simulink model "controller_stateflow"  (R2022b)
settings: Solver=FixedStepAuto  StartTime=0.0  StopTime=inf  FixedStep=0.05  RelTol=1e-3
PreLoadFcn:
  | rosinit();
model workspace (MAT data in the model file):
  SL_ROS_VariableLengthArrays_MaxSizes : object (value not decoded)
  pitch = -10
  restart = 0
undefined symbols (not defined in the file): StartTime
libraries: robotmaniplib x62, robotlib x17, robotcorelib x4, robotgazebolib x1
(part 4 of 4)

== stateflow chart controller_stateflow/General State Flow ==
  state Initialization0 [group]
    state initial_state
      entry:
      fprintf("Simulation started, setting initial conditions... ");
      sum_pos = [0;0;0];
      sum_ZYX = [0;0;0];
      send_command_ur10e = 0;
      send_command_panda = 0;
      send_command_sum = 0;
      panda_durTime = 2;
      ur_durTime = 2;
      state_velvet = 0;
      hand_state = 0.2;
      state_4 = 0;
      state_4_collBox = state_4;
      if pick_type<4
      state_4 = 2;
      end
    state initial_pose
      entry: fprintf("\n Go to home position...");
      [ur_pos,ur_durTime] = set_ur_initialState1();
      [panda_pos,panda_durTime] = set_panda_initialState();
      during:
      send_command_ur10e = 1;
      send_command_panda = 1;
      send_command_sum = 1;
    state Ready
      during: fprintf("--> Home position and initial poses done! \n");
      send_command_ur10e = 0;
      send_command_panda = 0;
      send_command_sum = 0;
      hand_state = 0.2;
    Initialization0.initial_state -> Initialization0.initial_pose : [controller_ready && link_state_ready]
    Initialization0.initial_pose -> Initialization0.Ready : [ur_finish && panda_finish && sum_finish]
  state Initialization [group]
    state initial_state
      entry:
      fprintf("Simulation started, setting initial conditions... ");
      sum_pos = [0;0;0];
      sum_ZYX = [0;0;0];
      send_command_ur10e = 0;
      send_command_panda = 0;
      send_command_sum = 0;
      panda_durTime = 2;
      ur_durTime = 2;
      state_velvet = 0;
      hand_state = 0.2;
      state_4 = 0;
      state_4_collBox = state_4;
      if pick_type<4
      state_4 = 2;
      end
    state initial_pose
      entry: fprintf("\n Go to home position...");
      [ur_pos,ur_durTime] = set_ur_initialState();
      [panda_pos,panda_durTime] = set_panda_initialState();
      during:
      send_command_ur10e = 1;
      send_command_panda = 1;
      send_command_sum = 1;
    state Ready
      entry: fprintf("--> Home position and initial poses done! \n");
      send_command_ur10e = 0;
      send_command_panda = 0;
      send_command_sum = 0;
      hand_state = 0.2;
    Initialization.initial_state -> Initialization.initial_pose : [controller_ready && link_state_ready]
    Initialization.initial_pose -> Initialization.Ready : [ur_finish && panda_finish && sum_finish]
  state [ur_pos,ur_durTime] = get_ur_pose4(box_pos,box_ZYX,box2_pos,box2_ZYX,sum_actual_pos,sum_actual_ZYX,ur_state,state) [function]
  state [ur_pos,durTime_ur] = get_ur_pose3(box_pose,box_ZYX,sum_actual_pos,sum_actual_ZYX,ur_state,state) [function]
  state [ur_pos,durTime_ur] = get_ur_pose(box_pose,box_ZYX,sum_actual_pos,sum_actual_ZYX,ur_state,state) [function]
  state [ur_pos,durTime_ur] = get_ur_pose2(box_pose,box_ZYX,sum_actual_pos,sum_actual_ZYX,ur_state,state) [function]
  state [panda_pos, panda_durTime] = get_panda_pose4(box_pos,box_ZYX,box2_pos,box2_ZYX,sum_actual_pos,sum_actual_ZYX,panda_state,state) [function]
  state [panda_pos,durTime_panda] = get_panda_pose3(box_pos,box_ZYX,sum_actual_pos,sum_actual_ZYX,panda_state,state) [function]
  state [panda_pos,durTime_panda] = get_panda_pose(box_pos,box_ZYX,sum_actual_pos,sum_actual_ZYX,panda_state,state) [function]
  state [panda_pos,durTime_panda] = get_panda_pose2(box_pos,box_ZYX,sum_actual_pos,sum_actual_ZYX,panda_state,state) [function]
  state Primitive_1 [group]
    state Going_near_the_pallet
      entry:
      fprintf("Picking type : 1 \n");
      fprintf("State 1: Going near the pallet... \n");
      during:
      distance_from_box = 0.8;
      distance_10 = 0.2;
      [sum_pos,sum_ZYX] = get_sum_pose_from_box(box_pos,box_ZYX,distance_from_box,distance_10,pick_type);
      send_command_sum = 1;
    state Setting_initial_arms_poses
      entry: fprintf("State 2: Setting initial arms poses... ");
      send_command_ur10e = 0;
      send_command_panda = 0;
      send_command_sum = 0;
      [ur_pos,ur_durTime] = get_ur_pose(box_pos,box_ZYX,sum_actual_pos,sum_actual_ZYX,ur_state,2);
      [panda_pos, panda_durTime] = get_panda_pose(box_pos,box_ZYX,sum_actual_pos,sum_actual_ZYX,panda_state,2);
      during:
      send_command_ur10e=1;
      send_command_panda = 1;
    state Going_near_the_box
      entry:fprintf("State 3: Going near the box... \n");
      send_command_panda = 0;
      send_command_sum = 0;
      distance_10 = 0;
      during:
      [sum_pos,sum_ZYX] = get_sum_pose_from_box(box_pos,box_ZYX,distance_from_box,distance_10,pick_type);
      send_command_sum = 1;
    state Softhand_goes_down
      entry: fprintf("State 4: Softhand goes down...\n");
      send_command_ur10e = 0;
      send_command_panda = 0;
      send_command_sum = 0;
      [ur_pos,ur_durTime] = get_ur_pose(box_pos,box_ZYX,sum_actual_pos,sum_actual_ZYX,ur_state,4);
      [panda_pos, panda_durTime]  = get_panda_pose(box_pos,box_ZYX,sum_actual_pos,sum_actual_ZYX,panda_state,4);
      during:
      send_command_panda = 1;
      send_command_ur10e = 1;
    state Getting_box_on_velvet
      entry: fprintf("State 5: Getting box on velvet...\n");
      send_command_panda = 0;
      send_command_ur10e = 0;
      [panda_pos, panda_durTime]  = get_panda_pose(box_pos,box_ZYX,sum_actual_pos,sum_actual_ZYX,panda_state,5);
      during:
      send_command_panda = 1;
      state_velvet = 1; %pick-up
    state Going_back_from_the_pallet_and_setting_holding_box_arms_poses
      entry: fprintf("State 7: Going back from the pallet...\n");
      fprintf("Setting holding box arms poses... ");
      distance_from_box = 0.8;
      distance_10 = 0.3;
      [sum_pos,sum_ZYX] = get_sum_pose_from_box(box_pos,box_ZYX,distance_from_box,distance_10,pick_type);
      send_command_ur10e = 0;
      send_command_panda = 0;
      send_command_sum = 0;
      [ur_pos,ur_durTime] = get_ur_pose(box_pos,box_ZYX,sum_actual_pos,sum_actual_ZYX,ur_state,7);
      [panda_pos, panda_durTime] = get_panda_pose(box_pos,box_ZYX,sum_actual_pos,sum_actual_ZYX,panda_state,7);
      during:
      send_command_sum = 1;
      send_command_ur10e=1;
      send_command_panda = 1;
    Primitive_1.Going_near_the_pallet -> Primitive_1.Setting_initial_arms_poses : [sum_finish && go>=2]
    Primitive_1.Setting_initial_arms_poses -> Primitive_1.Going_near_the_box : [ur_finish && panda_finish && go>=3]
    Primitive_1.Going_near_the_box -> Primitive_1.Softhand_goes_down : [sum_finish && go>=4]
    Primitive_1.Softhand_goes_down -> Primitive_1.Getting_box_on_velvet : [ur_finish && panda_finish && go>=5]{hand_state = 0.4;}
    Primitive_1.Getting_box_on_velvet -> Primitive_1.Going_back_from_the_pallet_and_setting_holding_box_arms_poses : [panda_finish && box_on_velvet && go>=6]{state_velvet = 0;}
  state Primitive_2 [group]
    state Going_near_the_pallet
      entry:
      fprintf("Picking type : 2 \n");
      fprintf("State 1: Going near the pallet... \n");
      during:
      distance_from_box = 0.85;
      distance_10 = 0.2;
      [sum_pos,sum_ZYX] = get_sum_pose_from_box(box_pos,box_ZYX,distance_from_box,distance_10,pick_type);
      send_command_sum = 1;
    state Setting_initial_arms_poses
      entry: fprintf("State 2: Setting initial arms poses... ");
      send_command_ur10e = 0;
      send_command_panda = 0;
      send_command_sum = 0;
      [ur_pos,ur_durTime] = get_ur_pose2(box_pos,box_ZYX,sum_actual_pos,sum_actual_ZYX,ur_state,2);
      [panda_pos, panda_durTime] = get_panda_pose2(box_pos,box_ZYX,sum_actual_pos,sum_actual_ZYX,panda_state,2);
      during:
      send_command_ur10e=1;
      send_command_panda = 1;
    state Going_near_the_box
      entry:fprintf("State 3: Going near the box... \n");
      send_command_panda = 0;
      send_command_sum = 0;
      distance_10 = 0;
      during:
      [sum_pos,sum_ZYX] = get_sum_pose_from_box(box_pos,box_ZYX,distance_from_box,distance_10,pick_type);
      send_command_sum = 1;
    state Softhand_goes_down
      entry: fprintf("State 4: Softhand goes down...\n");
      send_command_ur10e = 0;
      send_command_panda = 0;
      send_command_sum = 0;
      [panda_pos, panda_durTime]  = get_panda_pose2(box_pos,box_ZYX,sum_actual_pos,sum_actual_ZYX,panda_state,4);
      during:
      send_command_panda = 1;
    state Close_hand_and_approach_edge
      entry: fprintf("State 5: Close hand and approach edge...\n");
      send_command_panda = 0;
      hand_state = 0.6;
      [panda_pos, panda_durTime]  = get_panda_pose2(box_pos,box_ZYX,sum_actual_pos,sum_actual_ZYX,panda_state,5);
      during:
      send_command_panda = 1;
    state Getting_box_on_velvet
      entry: fprintf("State 6: Getting box on velvet...\n");
      send_command_panda = 0;
      [panda_pos, panda_durTime]  = get_panda_pose2(box_pos,box_ZYX,sum_actual_pos,sum_actual_ZYX,panda_state,6);
      during:
      send_command_panda = 1;
      %state_velvet = 1; %pick-up
    state Hand_up
      entry: fprintf("State 7: Hand up...\n");
      send_command_ur10e = 0;
      send_command_panda = 0;
      send_command_sum = 0;
      hand_state = 0.2;
      send_command_panda = 0;
      [panda_pos, panda_durTime]  = get_panda_pose2(box_pos,box_ZYX,sum_actual_pos,sum_actual_ZYX,panda_state,7);
      during:
      send_command_panda = 1;
    state Hand_reaches_the_lower_edge
      entry: fprintf("State 8: Hand reaches the lower edge...\n");
      send_command_panda = 0;
      [panda_pos, panda_durTime]  = get_panda_pose2(box_pos,box_ZYX,sum_actual_pos,sum_actual_ZYX,panda_state,8);
      during:
      send_command_panda = 1;
    state Hand_approaches_the_lower_edge
      entry: fprintf("State 9: Hand approaches the lower edge...\n");
      send_command_panda = 0;
      [panda_pos, panda_durTime]  = get_panda_pose2(box_pos,box_ZYX,sum_actual_pos,sum_actual_ZYX,panda_state,9);
      during:
      send_command_panda = 1;
    state Getting_the_box_aligned
      entry:
      entry: fprintf("State 10: Getting the box aligned...\n");
      send_command_ur10e = 0;
      send_command_panda = 0;
      send_command_sum = 0;
      sum_pos = sum_pos - [0;0.25;0];
      [ur_pos,ur_durTime] = get_ur_pose2(box_pos,box_ZYX,sum_actual_pos,sum_actual_ZYX,ur_state,10);
      [panda_pos, panda_durTime]  = get_panda_pose2(box_pos,box_ZYX,sum_actual_pos,sum_actual_ZYX,panda_state,10);
      during:
      send_command_ur10e=1;
      send_command_panda = 1;
      send_command_sum = 1;
    state Hand_approaches_the_lower_edge1
      entry: fprintf("State 11: Hand approaches the lower edge...\n");
      send_command_ur10e = 0;
      send_command_panda = 0;
      [panda_pos, panda_durTime]  = get_panda_pose2(box_pos,box_ZYX,sum_actual_pos,sum_actual_ZYX,panda_state,11);
      during:
      send_command_panda = 1;
    state Going_back_from_the_pallet_and_setting_holding_box_arms_poses
      entry: fprintf("State 12: Going back from the pallet...\n");
      fprintf("Settin holding box arms poses... ");
      distance_from_box = 0.8;
      distance_10 = 0.3;
      %[sum_pos,sum_ZYX] = get_sum_pose_from_box(box_pos,box_ZYX,distance_from_box,distance_10,pick_type);
      sum_pos = sum_pos - [0;0.5;0];
      send_command_ur10e = 0;
      send_command_panda = 0;
      send_command_sum = 0;
      [ur_pos,ur_durTime] = get_ur_pose(box_pos,box_ZYX,sum_actual_pos,sum_actual_ZYX,ur_state,7);
      [panda_pos, panda_durTime] = get_panda_pose(box_pos,box_ZYX,sum_actual_pos,sum_actual_ZYX,panda_state,7);
      during:
      send_command_sum = 1;
      send_command_ur10e=1;
      send_command_panda = 1;
    Primitive_2.Going_near_the_pallet -> Primitive_2.Setting_initial_arms_poses : [sum_finish && go>=2]
    Primitive_2.Setting_initial_arms_poses -> Primitive_2.Going_near_the_box : [ur_finish && panda_finish && go>=3]
    Primitive_2.Going_near_the_box -> Primitive_2.Softhand_goes_down : [sum_finish && go>=4]
    Primitive_2.Softhand_goes_down -> Close_hand_and_approach_edge : [panda_finish && go>=5]
    Close_hand_and_approach_edge -> Primitive_2.Getting_box_on_velvet : [panda_finish && go>=6]
    Primitive_2.Getting_box_on_velvet -> Hand_up : [panda_finish && box_on_velvet && go>=7]{state_velvet = 0;}
    Hand_up -> Hand_reaches_the_lower_edge : [panda_finish && go>=8]
    Hand_reaches_the_lower_edge -> Hand_approaches_the_lower_edge : [panda_finish && go>=9]
    Hand_approaches_the_lower_edge -> Getting_the_box_aligned : [panda_finish && go>=10]{hand_state = 0.6;}
    Getting_the_box_aligned -> Hand_approaches_the_lower_edge1 : [ur_finish && panda_finish && go>=11]{hand_state = 0.2;}
    Hand_approaches_the_lower_edge1 -> Primitive_2.Going_back_from_the_pallet_and_setting_holding_box_arms_poses : [panda_finish && go>=12]
  state Primitive_3 [group]
    state Going_near_the_pallet
      entry:
      fprintf("Picking type : 3 \n");
      fprintf("State 1: Going near the pallet... \n");
      during:
      distance_from_box = 0.85;
      distance_10 = 0.2;
      [sum_pos,sum_ZYX] = get_sum_pose_from_box(box_pos,box_ZYX,distance_from_box,distance_10,pick_type);
      send_command_sum = 1;
    state Setting_initial_arms_poses
      entry: fprintf("State 2: Setting initial arms poses... \n");
      send_command_ur10e = 0;
      send_command_panda = 0;
      send_command_sum = 0;
      [ur_pos,ur_durTime] = get_ur_pose3(box_pos,box_ZYX,sum_actual_pos,sum_actual_ZYX,ur_state,2);
      [panda_pos, panda_durTime] = get_panda_pose3(box_pos,box_ZYX,sum_actual_pos,sum_actual_ZYX,panda_state,2);
      during:
      send_command_ur10e=1;
      send_command_panda = 1;
    state Going_near_the_box
      entry:fprintf("State 3: Going near the box... \n");
      send_command_panda = 0;
      send_command_sum = 0;
      distance_10 = 0;
      during:
      [sum_pos,sum_ZYX] = get_sum_pose_from_box(box_pos,box_ZYX,distance_from_box,distance_10,pick_type);
      send_command_sum = 1;
    state Setting_initial_arms_poses_nearly
      entry: fprintf("State 4: Setting initial arms poses nearly... \n ");
      send_command_ur10e = 0;
      send_command_panda = 0;
      send_command_sum = 0;
      [ur_pos,ur_durTime] = get_ur_pose3(box_pos,box_ZYX,sum_actual_pos,sum_actual_ZYX,ur_state,4);
      [panda_pos, panda_durTime] = get_panda_pose3(box_pos,box_ZYX,sum_actual_pos,sum_actual_ZYX,panda_state,4);
      during:
      send_command_ur10e=1;
      send_command_panda = 1;
    state Softhand_goes_down
      entry: fprintf("State 5: Sofhand goes down...\n");
      send_command_ur10e = 0;
      send_command_panda = 0;
      [panda_pos, panda_durTime]  = get_panda_pose3(box_pos,box_ZYX,sum_actual_pos,sum_actual_ZYX,panda_state,5);
      during:
      send_command_panda = 1;
    state Softhand_reanches_and_approaches_the_edge
      entry: fprintf("State 6: Softhand reanches and approaches the edge, box up... \n");
      send_command_panda = 0;
      hand_state = 0.6;
      [panda_pos, panda_durTime]  = get_panda_pose3(box_pos,box_ZYX,sum_actual_pos,sum_actual_ZYX,panda_state,6);
      during:
      send_command_panda = 1;
    state Moving_Velvet_towards_the_box
      entry: fprintf("State 7: Moving Velvet towards the box... ");
      send_command_panda = 0;
      [ur_pos,ur_durTime] = get_ur_pose3(box_pos,box_ZYX,sum_actual_pos,sum_actual_ZYX,ur_state,7);
      during:
      send_command_ur10e = 1;
    state Moving_Velvet_under_the_box
      entry: fprintf("State 8: Moving Velvet under the box... ");
      send_command_ur10e = 0;
      [ur_pos,ur_durTime] = get_ur_pose3(box_pos,box_ZYX,sum_actual_pos,sum_actual_ZYX,ur_state,8);
      during:
      send_command_ur10e = 1;
    state Softhand_goes_far_from_box
      entry: fprintf("State 9: Softhand goes far from box...\n");
      send_command_panda = 0;
      send_command_ur10e = 0;
      [panda_pos, panda_durTime]  = get_panda_pose3(box_pos,box_ZYX,sum_actual_pos,sum_actual_ZYX,panda_state,9);
      during:
      send_command_panda = 1;
    state Getting_box_on_velvet
      entry: fprintf("State 10: Getting box on velvet, velvet on \n ");
      send_command_panda = 0;
      during:
      state_velvet = 1; %pick-up
    state Going_back_from_the_pallet_and_setting_holding_box_arms_poses
      entry: fprintf("State 11: Going back from the pallet...\n");
      fprintf("Settin holding box arms poses... ");
      distance_from_box = 1;
      distance_10 = 0.3;
      [sum_pos,sum_ZYX] = get_sum_pose_from_box(box_pos,box_ZYX,distance_from_box,distance_10,pick_type);
      send_command_ur10e = 0;
      send_command_panda = 0;
      send_command_sum = 0;
      [ur_pos,ur_durTime] = get_ur_pose3(box_pos,box_ZYX,sum_actual_pos,sum_actual_ZYX,ur_state,11);
      %[panda_pos, panda_durTime] = get_panda_pose3(box_pos,box_ZYX,sum_actual_pos,sum_actual_ZYX,panda_state,11);
      during:
      send_command_sum = 1;
      send_command_ur10e=1;
      %send_command_panda = 1;
    state Sofhand_goes_down
      entry: fprintf("State 12: Sofhand goes down ...\n");
      send_command_panda = 0;
      send_command_ur10e = 0;
      send_command_sum = 0;
      [panda_pos, panda_durTime]  = get_panda_pose3(box_pos,box_ZYX,sum_actual_pos,sum_actual_ZYX,panda_state,12);
      during:
      send_command_panda = 1;
    state Softhand_holding_box
      entry: fprintf("State 13: Sofhand holding box... \n");
      send_command_panda = 0;
      send_command_ur10e = 0;
      send_command_sum = 0;
      [panda_pos, panda_durTime]  = get_panda_pose3(box_pos,box_ZYX,sum_actual_pos,sum_actual_ZYX,panda_state,13);
      during:
      send_command_panda = 1;
      exit: hand_state = 0.4;
    Primitive_3.Going_near_the_pallet -> Primitive_3.Setting_initial_arms_poses : [sum_finish && go>=2]
    Primitive_3.Setting_initial_arms_poses -> Primitive_3.Going_near_the_box : [ur_finish && panda_finish && go>=3]
    Primitive_3.Going_near_the_box -> Setting_initial_arms_poses_nearly : [sum_finish && go>=4]
    Setting_initial_arms_poses_nearly -> Primitive_3.Softhand_goes_down : [ur_finish && panda_finish && go>=5]
    Primitive_3.Softhand_goes_down -> Softhand_reanches_and_approaches_the_edge : [panda_finish && go>=6]
    Softhand_reanches_and_approaches_the_edge -> Moving_Velvet_towards_the_box : [panda_finish && go>=7]
    Moving_Velvet_towards_the_box -> Moving_Velvet_under_the_box : [ur_finish && go>= 8]
    Moving_Velvet_under_the_box -> Softhand_goes_far_from_box : [ur_finish && go>=9]{ hand_state = 0.2;}
    Softhand_goes_far_from_box -> Primitive_3.Getting_box_on_velvet : [panda_finish && go >=10]
    Primitive_3.Getting_box_on_velvet -> Primitive_3.Going_back_from_the_pallet_and_setting_holding_box_arms_poses : [box_on_velvet]{state_velvet = 0;}
    Primitive_3.Going_back_from_the_pallet_and_setting_holding_box_arms_poses -> Sofhand_goes_down : [ur_finish && go>=12]
    Sofhand_goes_down -> Softhand_holding_box : [panda_finish && go>=13]
  state Primitive_4 [group]
    state Going_near_the_pallet
      entry:
      fprintf("Picking type : 4 \n");
      fprintf("State 1: Going near the pallet... \n");
      during:
      distance_from_box = 0.8;
      distance_10 = 0.2;
      [sum_pos,sum_ZYX] = get_sum_pose_from_box4(box_pos,box_ZYX,box2_pos,box2_ZYX,distance_from_box,distance_10,state_4);
      send_command_sum = 1;
    state Open_both_hands2
      entry: fprintf("Picking Strategy for the second box. \n");
      fprintf("State 2: Open both hands... ");
      send_command_ur10e = 0;
      send_command_panda = 0;
      send_command_sum = 0;
      [ur_pos,ur_durTime] = get_ur_pose4(box_pos,box_ZYX,box2_pos,box2_ZYX,sum_actual_pos,sum_actual_ZYX,ur_state,102);
      [panda_pos, panda_durTime] = get_panda_pose4(box_pos,box_ZYX,box2_pos,box2_ZYX,sum_actual_pos,sum_actual_ZYX,panda_state,102);
      during:
      send_command_ur10e=1;
      send_command_panda = 1;
    state Open_both_hands
      entry: fprintf("Picking Strategy for the first box. \n");
      fprintf("State 2: Open both hands... ");
      send_command_ur10e = 0;
      send_command_panda = 0;
      send_command_sum = 0;
      [ur_pos,ur_durTime] = get_ur_pose4(box_pos,box_ZYX,box2_pos,box2_ZYX,sum_actual_pos,sum_actual_ZYX,ur_state,101);
      [panda_pos, panda_durTime] = get_panda_pose4(box_pos,box_ZYX,box2_pos,box2_ZYX,sum_actual_pos,sum_actual_ZYX,panda_state,101);
      during:
      send_command_ur10e=1;
      send_command_panda = 1;
    state Going_near_the_box2
      entry:fprintf("State 3: Going near the box... \n");
      distance_10 = 0;
      during:
      [sum_pos,sum_ZYX] = get_sum_pose_from_box4(box_pos,box_ZYX,box2_pos,box2_ZYX,distance_from_box,distance_10,state_4);
      send_command_sum = 1;
    state Going_near_the_box
      entry:fprintf("State 3: Going near the box... \n");
      distance_10 = 0;
      during:
      [sum_pos,sum_ZYX] = get_sum_pose_from_box4(box_pos,box_ZYX,box2_pos,box2_ZYX,distance_from_box,distance_10,state_4);
      send_command_sum = 1;
    state Hold_both_boxes
      entry: fprintf("State 4: Hold both boxes... ");
      send_command_ur10e = 0;
      send_command_panda = 0;
      send_command_sum = 0;
      [ur_pos,ur_durTime] = get_ur_pose4(box_pos,box_ZYX,box2_pos,box2_ZYX,sum_actual_pos,sum_actual_ZYX,ur_state,111);
      [panda_pos, panda_durTime] = get_panda_pose4(box_pos,box_ZYX,box2_pos,box2_ZYX,sum_actual_pos,sum_actual_ZYX,panda_state,111);
      during:
      send_command_ur10e=1;
      send_command_panda = 1;
    state Hold_both_boxes2
      entry: fprintf("State 4: Hold both boxes... ");
      send_command_ur10e = 0;
      send_command_panda = 0;
      send_command_sum = 0;
      [ur_pos,ur_durTime] = get_ur_pose4(box_pos,box_ZYX,box2_pos,box2_ZYX,sum_actual_pos,sum_actual_ZYX,ur_state,112);
      [panda_pos, panda_durTime] = get_panda_pose4(box_pos,box_ZYX,box2_pos,box2_ZYX,sum_actual_pos,sum_actual_ZYX,panda_state,112);
      during:
      send_command_ur10e=1;
      send_command_panda = 1;
    state Rotate_first_box
      entry: fprintf("State 5: Rotate first box... ");
      send_command_ur10e = 0;
      send_command_panda = 0;
      [panda_pos, panda_durTime]  = get_panda_pose4(box_pos,box_ZYX,box2_pos,box2_ZYX,sum_actual_pos,sum_actual_ZYX,panda_state,121);
      during:
      send_command_panda = 1;
    state Rotate_second_box
      entry: fprintf("State 5: Rotate second box... ");
      send_command_panda = 0;
      send_command_ur10e = 0;
      hand_state = 0.5;
      [ur_pos,ur_durTime] = get_ur_pose4(box_pos,box_ZYX,box2_pos,box2_ZYX,sum_actual_pos,sum_actual_ZYX,ur_state,122);
      [panda_pos, panda_durTime]  = get_panda_pose4(box_pos,box_ZYX,box2_pos,box2_ZYX,sum_actual_pos,sum_actual_ZYX,panda_state,122);
      during:
      send_command_panda = 1;
      send_command_ur10e = 1;
    state Reopen_both_arms1
      entry: fprintf("State 6: Reopen both arms.. ");
      send_command_panda = 0;
      send_command_ur10e = 0;
      hand_state = 0.2;
      [ur_pos,ur_durTime] = get_ur_pose4(box_pos,box_ZYX,box2_pos,box2_ZYX,sum_actual_pos,sum_actual_ZYX,ur_state,132);
      [panda_pos, panda_durTime]  = get_panda_pose4(box_pos,box_ZYX,box2_pos,box2_ZYX,sum_actual_pos,sum_actual_ZYX,panda_state,132);
      during:
      send_command_panda = 1;
      send_command_ur10e=1;
    state Reopen_both_arms
      entry: fprintf("State 6: Reopen both arms.. ");
      send_command_panda = 0;
      send_command_ur10e = 0;
      [ur_pos,ur_durTime] = get_ur_pose4(box_pos,box_ZYX,box2_pos,box2_ZYX,sum_actual_pos,sum_actual_ZYX,ur_state,131);
      [panda_pos, panda_durTime]  = get_panda_pose4(box_pos,box_ZYX,box2_pos,box2_ZYX,sum_actual_pos,sum_actual_ZYX,panda_state,131);
      during:
      send_command_panda = 1;
      send_command_ur10e=1;
    Primitive_4.Going_near_the_pallet -> Open_both_hands [order 1] : [sum_finish && state_4 == 1 && go>=2]
    Primitive_4.Going_near_the_pallet -> Open_both_hands2 [order 2] : [sum_finish && state_4 == 2 && go>=2]
    Open_both_hands2 -> Going_near_the_box2 : [ur_finish && panda_finish && go>=3]
    Open_both_hands -> Primitive_4.Going_near_the_box : [ur_finish && panda_finish && go>=3]
    Primitive_4.Going_near_the_box -> Hold_both_boxes : [sum_finish && go>=4]
    Going_near_the_box2 -> Hold_both_boxes2 : [sum_finish && go>=4]
    Hold_both_boxes -> Rotate_first_box : [ur_finish && panda_finish && go>=5]
    Hold_both_boxes2 -> Rotate_second_box : [ur_finish && panda_finish && go>=5]
    Rotate_first_box -> Reopen_both_arms : [panda_finish && go>=6]
    Rotate_second_box -> Reopen_both_arms1 : [ur_finish && panda_finish && go>=6]
  state Primitive_1_for_piking_type_4 [group]
    state Going_near_the_pallet
      entry:
      fprintf("Picking type : 1 \n");
      fprintf("State 1: Going near the pallet... \n");
      during:
      distance_from_box = 0.8;
      distance_10 = 0.2;
      [sum_pos,sum_ZYX] = get_sum_pose_from_box(box_pos,box_ZYX,distance_from_box,distance_10,pick_type);
      send_command_sum = 1;
    state Going_near_the_pallet1
      entry:
      fprintf("Picking type : 1 \n");
      fprintf("State 1: Going near the pallet... \n");
      during:
      distance_from_box = 0.8;
      distance_10 = 0.2;
      [sum_pos,sum_ZYX] = get_sum_pose_from_box(box2_pos,box2_ZYX,distance_from_box,distance_10,pick_type);
      send_command_sum = 1;
    state Setting_initial_arms_poses
      entry: fprintf("State 2: Setting initial arms poses... ");
      send_command_ur10e = 0;
      send_command_panda = 0;
      send_command_sum = 0;
      [ur_pos,ur_durTime] = get_ur_pose(box_pos,box_ZYX,sum_actual_pos,sum_actual_ZYX,ur_state,2);
      [panda_pos, panda_durTime] = get_panda_pose(box_pos,box_ZYX,sum_actual_pos,sum_actual_ZYX,panda_state,2);
      during:
      send_command_ur10e=1;
      send_command_panda = 1;
    state Setting_initial_arms_poses1
      entry: fprintf("State 2: Setting initial arms poses... ");
      send_command_ur10e = 0;
      send_command_panda = 0;
      send_command_sum = 0;
      [ur_pos,ur_durTime] = get_ur_pose(box2_pos,box2_ZYX,sum_actual_pos,sum_actual_ZYX,ur_state,2);
      [panda_pos, panda_durTime] = get_panda_pose(box2_pos,box2_ZYX,sum_actual_pos,sum_actual_ZYX,panda_state,2);
      during:
      send_command_ur10e=1;
      send_command_panda = 1;
    state Going_near_the_box
      entry:fprintf("State 3: Going near the box... \n");
      send_command_panda = 0;
      send_command_sum = 0;
      distance_10 = 0;
      during:
      [sum_pos,sum_ZYX] = get_sum_pose_from_box(box_pos,box_ZYX,distance_from_box,distance_10,pick_type);
      send_command_sum = 1;
    state Going_near_the_box1
      entry:fprintf("State 3: Going near the box... \n");
      send_command_panda = 0;
      send_command_sum = 0;
      distance_10 = 0;
      during:
      [sum_pos,sum_ZYX] = get_sum_pose_from_box(box2_pos,box2_ZYX,distance_from_box,distance_10,pick_type);
      send_command_sum = 1;
    state Softhand_goes_down
      entry: fprintf("State 4: Softhand goes down...\n");
      send_command_ur10e = 0;
      send_command_panda = 0;
      send_command_sum = 0;
      [ur_pos,ur_durTime] = get_ur_pose(box_pos,box_ZYX,sum_actual_pos,sum_actual_ZYX,ur_state,4);
      [panda_pos, panda_durTime]  = get_panda_pose(box_pos,box_ZYX,sum_actual_pos,sum_actual_ZYX,panda_state,4);
      during:
      send_command_panda = 1;
      send_command_ur10e = 1;
    state Softhand_goes_down1
      entry: fprintf("State 4: Softhand goes down...\n");
      send_command_ur10e = 0;
      send_command_panda = 0;
      send_command_sum = 0;
      [ur_pos,ur_durTime] = get_ur_pose(box2_pos,box2_ZYX,sum_actual_pos,sum_actual_ZYX,ur_state,4);
      [panda_pos, panda_durTime]  = get_panda_pose(box2_pos,box2_ZYX,sum_actual_pos,sum_actual_ZYX,panda_state,4);
      during:
      send_command_panda = 1;
      send_command_ur10e = 1;
    state Getting_box_on_velvet
      entry: fprintf("State 5: Getting box on velvet...\n");
      send_command_panda = 0;
      send_command_ur10e = 0;
      [panda_pos, panda_durTime]  = get_panda_pose(box_pos,box_ZYX,sum_actual_pos,sum_actual_ZYX,panda_state,5);
      during:
      send_command_panda = 1;
      state_velvet = 1; %pick-up
    state Getting_box_on_velvet1
      entry: fprintf("State 5: Getting box on velvet...\n");
      send_command_panda = 0;
      send_command_ur10e = 0;
      [panda_pos, panda_durTime]  = get_panda_pose(box2_pos,box2_ZYX,sum_actual_pos,sum_actual_ZYX,panda_state,5);
      during:
      send_command_panda = 1;
      state_velvet = 1; %pick-up
    state Hold_box_on_velvet
      entry: fprintf("State 6: Hold box on velvet...\n");
      send_command_panda = 0;
      [panda_pos, panda_durTime]  = get_panda_pose(box_pos,box_ZYX,sum_actual_pos,sum_actual_ZYX,panda_state,6);
      during:
      send_command_panda = 1;
    state Hold_box_on_velvet1
      entry: fprintf("State 6: Hold box on velvet...\n");
      send_command_panda = 0;
      [panda_pos, panda_durTime]  = get_panda_pose(box2_pos,box2_ZYX,sum_actual_pos,sum_actual_ZYX,panda_state,6);
      during:
      send_command_panda = 1;
    state Going_back_from_the_pallet_and_setting_holding_box_arms_poses
      entry: fprintf("State 7: Going back from the pallet...\n");
      fprintf("Setting holding box arms poses... ");
      distance_from_box = 0.8;
      distance_10 = 0.3;
      [sum_pos,sum_ZYX] = get_sum_pose_from_box(box_pos,box_ZYX,distance_from_box,distance_10,pick_type);
      send_command_ur10e = 0;
      send_command_panda = 0;
      send_command_sum = 0;
      [ur_pos,ur_durTime] = get_ur_pose(box_pos,box_ZYX,sum_actual_pos,sum_actual_ZYX,ur_state,7);
      [panda_pos, panda_durTime] = get_panda_pose(box_pos,box_ZYX,sum_actual_pos,sum_actual_ZYX,panda_state,7);
      during:
      send_command_sum = 1;
      send_command_ur10e=1;
      send_command_panda = 1;
    state Going_back_from_the_pallet_and_setting_holding_box_arms_poses1
      entry: fprintf("State 7: Going back from the pallet...\n");
      fprintf("Setting holding box arms poses... ");
      distance_from_box = 0.8;
      distance_10 = 0.3;
      [sum_pos,sum_ZYX] = get_sum_pose_from_box(box2_pos,box2_ZYX,distance_from_box,distance_10,pick_type);
      send_command_ur10e = 0;
      send_command_panda = 0;
      send_command_sum = 0;
      [ur_pos,ur_durTime] = get_ur_pose(box2_pos,box2_ZYX,sum_actual_pos,sum_actual_ZYX,ur_state,7);
      [panda_pos, panda_durTime] = get_panda_pose(box2_pos,box2_ZYX,sum_actual_pos,sum_actual_ZYX,panda_state,7);
      during:
      send_command_sum = 1;
      send_command_ur10e=1;
      send_command_panda = 1;
    Primitive_1_for_piking_type_4.Going_near_the_pallet -> Primitive_1_for_piking_type_4.Setting_initial_arms_poses : [sum_finish && go>=8]
    Going_near_the_pallet1 -> Setting_initial_arms_poses1 : [sum_finish && go>=8]
    Primitive_1_for_piking_type_4.Setting_initial_arms_poses -> Primitive_1_for_piking_type_4.Going_near_the_box : [ur_finish && panda_finish && go>=9]
    Setting_initial_arms_poses1 -> Going_near_the_box1 : [ur_finish && panda_finish && go>=9]
    Primitive_1_for_piking_type_4.Going_near_the_box -> Primitive_1_for_piking_type_4.Softhand_goes_down : [sum_finish && go>=10]
    Going_near_the_box1 -> Softhand_goes_down1 : [sum_finish && go>=10]
    Primitive_1_for_piking_type_4.Softhand_goes_down -> Primitive_1_for_piking_type_4.Getting_box_on_velvet : [ur_finish && panda_finish && go>=11]{hand_state = 0.4;}
    Softhand_goes_down1 -> Getting_box_on_velvet1 : [ur_finish && panda_finish && go>=11]{hand_state = 0.4;}
    Primitive_1_for_piking_type_4.Getting_box_on_velvet -> Primitive_1_for_piking_type_4.Going_back_from_the_pallet_and_setting_holding_box_arms_poses : [panda_finish && box_on_velvet && go>=12]{state_velvet = 0;}
    Getting_box_on_velvet1 -> Going_back_from_the_pallet_and_setting_holding_box_arms_poses1 : [panda_finish && box_on_velvet && go>=12]{state_velvet = 0;}
    Hold_box_on_velvet -> Primitive_1_for_piking_type_4.Going_back_from_the_pallet_and_setting_holding_box_arms_poses : [panda_finish && go>=13]
    Hold_box_on_velvet1 -> Going_back_from_the_pallet_and_setting_holding_box_arms_poses1 : [panda_finish && go>=13]
  state Return home with box [group]
    state Go_back
      entry: fprintf("Picking phase completed! \n");
      fprintf("Return home position... \n");
      send_command_sum = 0;
      send_command_ur10e = 0;
      send_command_panda = 0;
      during:
      sum_pos = [0;0;0];
      sum_ZYX = [0;0;0];
      send_command_sum = 1;
    state finish
      entry: fprintf("Home position reached...\n");
      send_command_sum = 0;
    Go_back -> Return.finish : [sum_finish]
  state [ur_pos,durTime_ur] = get_ur_pose_cnvy(tra_pos,tra_ZYX,sum_actual_pos,sum_actual_ZYX,ur_state,state) [function]
  state [panda_pos,durTime_panda] = get_panda_pose_cnvy(tra_pos,tra_ZYX,sum_actual_pos,sum_actual_ZYX,panda_state,state) [function]
  state Release [group]
    state Go_near_the_conveyor_belt
      entry : fprintf("Release Phase: \n");
      fprintf("Go near the conveyor belt ... \n");
      during:
      distance_from_cnvy = 0.8;
      [sum_pos,sum_ZYX] = get_sum_pose_from_cnvy(tra_pos,tra_ZYX,distance_from_cnvy);
      send_command_sum = 1;
    state Franka_Hand_up
      entry: fprintf("Franka Hand Up... \n");
      send_command_ur10e = 0;
      send_command_panda = 0;
      send_command_sum = 0;
      [panda_pos, panda_durTime] = get_panda_pose_cnvy(box_pos,box_ZYX,sum_actual_pos,sum_actual_ZYX,panda_state,93);
      during:
      send_command_panda = 1;
    state Align_UR_Velvet
      entry: fprintf("Align UR Velvet... \n");
      send_command_ur10e = 0;
      send_command_panda = 0;
      send_command_sum = 0;
      [ur_pos,ur_durTime] = get_ur_pose_cnvy(tra_pos,tra_ZYX,sum_actual_pos,sum_actual_ZYX,ur_state,1);
      during:
      send_command_ur10e = 1;
    state Pull_out_box
      entry: fprintf("Box Off... \n");
      during:
      state_velvet = -1; %pick-off
    state Go_back_from_the_conveyor_belt
      entry: fprintf("Release phase completed! \n");
      fprintf("Go back from the conveyor belt... \n");
      send_command_ur10e = 0;
      send_command_panda = 0;
      send_command_sum = 0;
      during:
      distance_from_cnvy = 0.8;
      [sum_pos,sum_ZYX] = get_sum_pose_from_cnvy(tra_pos,tra_ZYX,distance_from_cnvy);
      send_command_sum = 1;
    Go_near_the_conveyor_belt -> Franka_Hand_up : [sum_finish && go>21]
    Franka_Hand_up -> Align_UR_Velvet : [panda_finish && go>22]
    Align_UR_Velvet -> Pull_out_box : [ur_finish  && go>23]
    Pull_out_box -> Go_back_from_the_conveyor_belt : [box_off && go>24]{state_velvet = 0;}
  state Finish [group]
    state Return_home
      entry:
      fprintf("Return home position... \n");
      send_command_sum = 0;
      during:
      sum_pos = [0;0;0];
      sum_ZYX = [0;0;0];
      [ur_pos,ur_durTime] = set_ur_initialState();
      [panda_pos,panda_durTime] = set_panda_initialState();
      send_command_ur10e = 1;
      send_command_panda = 1;
      send_command_sum = 1;
    state finish
      entry: fprintf(" --- Mission Completed ! --- \n");
      send_command_ur10e = 0;
      send_command_panda = 0;
      send_command_sum = 0;
    Return_home -> Finish.finish : [ur_finish && panda_finish && sum_finish]
  state THE_END
  (default) -> Initialization0.initial_state
  Initialization0.Ready -> Initialization.initial_state : [go > 1]
  Go_back_from_the_conveyor_belt -> Initialization.initial_pose [order 1] : [sum_finish && go>16 && state_4 == 1]
  Initialization.Ready -> Primitive_4.Going_near_the_pallet [order 3] : [pick_type == 4 && go>=1]{state_4 = state_4 +1; state_4_collBox = state_4;}
  Initialization.Ready -> Primitive_1.Going_near_the_pallet [order 2] : [pick_type == 1 && go>=1]
  Initialization.Ready -> Primitive_2.Going_near_the_pallet [order 1] : [pick_type == 2 && go>=1]
  Initialization.Ready -> Primitive_3.Going_near_the_pallet [order 4] : [pick_type == 3 && go>=1]
  Reopen_both_arms -> Primitive_1_for_piking_type_4.Going_near_the_pallet : [ur_finish && panda_finish && go>=7]
  Reopen_both_arms1 -> Going_near_the_pallet1 : [ur_finish && panda_finish && go>=7]
  Primitive_1.Going_back_from_the_pallet_and_setting_holding_box_arms_poses -> Go_back : [sum_finish && go>=8]
  Primitive_2.Going_back_from_the_pallet_and_setting_holding_box_arms_poses -> Go_back : [sum_finish && go>=13]
  Softhand_holding_box -> Go_back : [panda_finish && go>=14]
  Primitive_1_for_piking_type_4.Going_back_from_the_pallet_and_setting_holding_box_arms_poses -> Go_back : [sum_finish && go>14]
  Going_back_from_the_pallet_and_setting_holding_box_arms_poses1 -> Go_back : [sum_finish && go>14]
  Return.finish -> Go_near_the_conveyor_belt : [go>20]
  Go_back_from_the_conveyor_belt -> Return_home [order 2] : [sum_finish && go>25 && state_4 == 2]
  Finish.finish -> THE_END
  data: ur_Pos function_output; ur_durTime_ function_output; ur_Pos function_output; ur_durTime_ function_output; panda_pos function_output; panda_durTime_ function_output; sum_pos function_output; sum_ZYX function_output; box_pos function_input; box_ZYX function_input; distance_from_box function_input; distance_10 function_input; pick_type function_input; sum_pos function_output; sum_ZYX function_output; box_pos function_input; box_ZYX function_input; box2_pos function_input; box2_ZYX function_input; distance_from_box function_input; distance_10 function_input; state_4 function_input; box_pos function_input double size=[3,1]; box_ZYX function_input double size=[3,1]; box2_pos function_input double size=[3,1]; box2_ZYX function_input double size=[3,1]; sum_actual_pos function_input double size=[3,1]; sum_actual_ZYX function_input double size=[3,1]; ur_state function_input double size=[7,1]; ur_pos function_output; ur_durTime function_output; state function_input double size=1; box_pose function_input double size=[3,1]; box_ZYX function_input double size=[3,1]; sum_actual_pos function_input double size=[3,1]; sum_actual_ZYX function_input double size=[3,1]; ur_state function_input double size=[7,1]; ur_pos function_output; state function_input double size=1; durTime_ur function_output; box_pose function_input double size=[3,1]; box_ZYX function_input double size=[3,1]; sum_actual_pos function_input double size=[3,1]; sum_actual_ZYX function_input double size=[3,1]; ur_state function_input double size=[7,1]; ur_pos function_output; state function_input double size=1; durTime_ur function_output; box_pose function_input double size=[3,1]; box_ZYX function_input double size=[3,1]; sum_actual_pos function_input double size=[3,1]; sum_actual_ZYX function_input double size=[3,1]; ur_state function_input double size=[7,1]; ur_pos function_output; state function_input double size=1; durTime_ur function_output; box_pos function_input double size=[3,1]; box_ZYX function_input double size=[3,1]; box2_pos function_input double size=[3,1]; box2_ZYX function_input double size=[3,1]; sum_actual_pos function_input double size=[3,1]; sum_actual_ZYX function_input double size=[3,1]; panda_state function_input double size=[7,1]; panda_pos function_output; panda_durTime function_output; state function_input double size=1; box_pos function_input double size=[3,1]; box_ZYX function_input double size=[3,1]; sum_actual_pos function_input double size=[3,1]; sum_actual_ZYX function_input double size=[3,1]; panda_state function_input double size=[7,1]; panda_pos function_output; state function_input double size=1; durTime_panda function_output; box_pos function_input double size=[3,1]; box_ZYX function_input double size=[3,1]; sum_actual_pos function_input double size=[3,1]; sum_actual_ZYX function_input double size=[3,1]; panda_state function_input double size=[7,1]; panda_pos function_output; state function_input double size=1; durTime_panda function_output; box_pos function_input double size=[3,1]; box_ZYX function_input double size=[3,1]; sum_actual_pos function_input double size=[3,1]; sum_actual_ZYX function_input double size=[3,1]; panda_state function_input double size=[7,1]; panda_pos function_output; state function_input double size=1; durTime_panda function_output; sum_pos function_output; sum_ZYX function_output; tra_pos function_input; tra_ZYX function_input; distance_from_cnvy function_input; tra_pos function_input double size=[3,1]; tra_ZYX function_input double size=[3,1]; sum_actual_pos function_input double size=[3,1]; sum_actual_ZYX function_input double size=[3,1]; ur_state function_input double size=[7,1]; state function_input double size=1; ur_pos function_output; durTime_ur function_output; tra_pos function_input double size=[3,1]; tra_ZYX function_input double size=[3,1]; sum_actual_pos function_input double size=[3,1]; sum_actual_ZYX function_input double size=[3,1]; panda_state function_input double size=[7,1]; panda_pos function_output; state function_input double size=1; durTime_panda function_output; sf_internal_action_state_placeholder_data local double size=1 =0; pick_type input; send_command_ur10e output size=1,1; controller_ready input; link_state_ready input; go input; send_command_panda output size=1,1; send_command_sum output size=1,1; ur_pos output size=[6,5]; ur_durTime output size=1; panda_pos output; panda_durTime output size=1; sum_pos output; panda_state input; ur_state input; sum_actual_pos input; sum_actual_ZYX input; panda_finish input; sum_finish input; ur_finish input; box_pos input; box_ZYX input; sum_ZYX output; distance_10 local; distance_from_box local; box_on_velvet input; box_off input; box2_pos input size=[3,1]; box2_ZYX input size=[3,1]; tra_ZYX input; tra_pos input; state_velvet output size=1; hand_state output; state_4 local; state_4_collBox output size=1; distance_from_cnvy local
  function [ur_Pos,ur_durTime_]= set_ur_initialState1:
    | function [ur_Pos,ur_durTime_]= set_ur_initialState1
    | % Set initial pose of UR Manipulator
    | 
    |     
    |     ur_pos_  = ([0 -90 0 0 0 0]').*pi/180;
    | 
    |     ur_Pos = horzcat(ur_pos_,ur_pos_,ur_pos_,ur_pos_,ur_pos_);
    |     ur_durTime_ = 3;
    | end
  function [ur_Pos,ur_durTime_]= set_ur_initialState:
    | function [ur_Pos,ur_durTime_]= set_ur_initialState
    | % Set initial pose of UR Manipulator
    | 
    |     ur_pos_  = [-0.6416,-5.6222+2*pi,-2.4013,-4.5429+2*pi,0.9292,-3.1416]';
    |     ur_pos_  = ([-90-71.37,-102.78,-141.66,-70.64,-62.79,-205.96]').*pi/180;
    | 
    |     ur_Pos = horzcat(ur_pos_,ur_pos_,ur_pos_,ur_pos_,ur_pos_);
    |     ur_durTime_ = 3;
    | end
  function [panda_pos,panda_durTime_] = set_panda_initialState:
    | function [panda_pos,panda_durTime_] = set_panda_initialState
    | % Set initial pose of Panda Manipulator
    |  panda_pos_ = [0;-0.7853;0;-2.35619;0;1.57079;0.785398];
    |  panda_pos = horzcat(panda_pos_,panda_pos_,panda_pos_,panda_pos_,panda_pos_);
    |  panda_durTime_ = 3;
    | end
  function [sum_pos,sum_ZYX] = get_sum_pose_from_box(box_pos,box_ZYX,distance_from_box,distance_10,pick_type):
    | function [sum_pos,sum_ZYX] = get_sum_pose_from_box(box_pos,box_ZYX,distance_from_box,distance_10,pick_type)
    |     
    |     base_sum_length = 0.75; 
    |     sum_pos = [0;0;0];
    |     sum_ZYX = [0;0;0];
    |     % questo mi calcola la posizione in cui deve andare il robot, partendo
    |     % dalla posizione del box e aggiungendo un vettore distanza verso
    |     % l'asse y negativo del box
    |     if pick_type == 1 || pick_type == 2
    |         back_from_box = box_pos + [eul2rotm(box_ZYX', 'ZYX')]*[0; -distance_from_box - distance_10 - base_sum_length/2;0];
    |         sum_pos = [back_from_box(1);back_from_box(2);0];
    | 
    |         % l'orientazione è solo relativa alla posa della scatola sul piano XY
    |         % ed è solo ruotata di 90 gradi
    |         sum_ZYX = [box_ZYX(1)+pi/2;0;0];  
    |     end
    |     if pick_type == 3
    |         back_from_box = box_pos +[0.115;0.115;0.065] + [eul2rotm(box_ZYX', 'ZYX')]*[0; distance_from_box + distance_10 + base_sum_length/2;0];
    |         sum_pos = [back_from_box(1);back_from_box(2);0];
    |     
    |         % l'orientazione è solo relativa alla posa della scatola sul piano XY
    |         % ed è solo ruotata di 90 gradi
    |         sum_ZYX = [box_ZYX(1)-pi/2;0;0];  
    |     end
    |     if pick_type == 4
    |         back_from_box = box_pos + [eul2rotm(box_ZYX', 'ZYX')]*[-0.38/2; -distance_from_box - distance_10 - base_sum_length/2;0];
    |         sum_pos = [back_from_box(1);back_from_box(2);0];
    | 
    |         % l'orientazione è solo relativa alla posa della scatola sul piano XY
    |         % ed è solo ruotata di 90 gradi
    |         sum_ZYX = [box_ZYX(1)+pi/2;0;0];  
    |     end
    | end
  function [sum_pos,sum_ZYX] = get_sum_pose_from_box4(box_pos,box_ZYX,box2_pos,box2_ZYX,distance_from_box,distance_10,state_4):
    | function [sum_pos,sum_ZYX] = get_sum_pose_from_box4(box_pos,box_ZYX,box2_pos,box2_ZYX,distance_from_box,distance_10,state_4)
    |     
    |     base_sum_length = 0.75; 
    |     sum_pos = [0;0;0];
    |     sum_ZYX = [0;0;0];
    |     % questo mi calcola la posizione in cui deve andare il robot, partendo
    |     % dalla posizione del box e aggiungendo un vettore distanza verso
    |     % l'asse y negativo del box
    | 
    |     if state_4 == 1
    |         back_from_box = box_pos + [eul2rotm(box_ZYX', 'ZYX')]*[-0.38/2; -distance_from_box - distance_10 - base_sum_length/2;0];
    |         sum_pos = [back_from_box(1);back_from_box(2);0];
    | 
    |         % l'orientazione è solo relativa alla posa della scatola sul piano XY
    |         % ed è solo ruotata di 90 gradi
    |         sum_ZYX = [box_ZYX(1)+pi/2;0;0];  
    |     end
    |     if state_4 == 2
    |         back_from_box = box2_pos + [eul2rotm(box2_ZYX', 'ZYX')]*[0; -distance_from_box - distance_10 - base_sum_length/2;0];
    |         sum_pos = [back_from_box(1);back_from_box(2);0];
    | 
    |         % l'orientazione è solo relativa alla posa della scatola sul piano XY
    |         % ed è solo ruotata di 90 gradi
    |         sum_ZYX = [box2_ZYX(1)+pi/2;0;0];  
    |     end    
    | end
  function [sum_pos,sum_ZYX] = get_sum_pose_from_cnvy(tra_pos,tra_ZYX,distance_from_cnvy):
    | function [sum_pos,sum_ZYX] = get_sum_pose_from_cnvy(tra_pos,tra_ZYX,distance_from_cnvy)
    |     
    |     base_sum_length = 0.75;         
    |     traDim = [1;5.456930;0.192575];
    | 
    |     back_from_box = tra_pos + [eul2rotm(tra_ZYX', 'ZYX')]*[0; traDim(2)/2 + distance_from_cnvy + base_sum_length/2;0];
    |     
    |     sum_pos = [back_from_box(1);back_from_box(2);0];
    |     sum_ZYX = [tra_ZYX(1)-pi/2;0;0];  
    | 
    |         
    | end
